simulink model "DragModelSeparateRotors"  (R2015b)
settings: Solver=VariableStepAuto  StartTime=0.0  StopTime=10.0  RelTol=1e-3
settings Model: Creator=jban039  LastModifiedBy=jban039

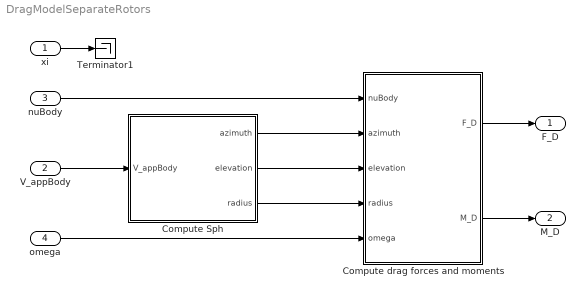
== system DragModelSeparateRotors ==
  xi : Inport  PortDimensions=3
  V_appBody : Inport  Port=2  PortDimensions=3
  nuBody : Inport  Port=3  PortDimensions=3
  omega : Inport  Port=4  PortDimensions=Uav.N_ROTORS
  Compute Sph : MATLAB Function  TreatAsAtomicUnit=on
  Compute drag forces and moments : MATLAB Function  TreatAsAtomicUnit=on
  Terminator1 : Terminator
  F_D : Outport
  M_D : Outport  Port=2
  wires:
  Compute drag forces and moments/1(F_D) -> F_D/1
  Compute drag forces and moments/2(M_D) -> M_D/1
  xi/1 -> Terminator1/1
  omega/1 -> Compute drag forces and moments/5(omega)
  nuBody/1 -> Compute drag forces and moments/1(nuBody)
  V_appBody/1 -> Compute Sph/1(V_appBody)
  Compute Sph/3(radius) -> Compute drag forces and moments/4(radius)
  Compute Sph/2(elevation) -> Compute drag forces and moments/3(elevation)
  Compute Sph/1(azimuth) -> Compute drag forces and moments/2(azimuth)

== matlab function DragModelSeparateRotors/Compute Sph ==
  data: V_appBody input; azimuth output; elevation output; radius output
function [azimuth, elevation, radius] = computeSph(V_appBody)
%#codegen

% Convert from polar to spherical coordinates
[ azimuth, elevation, radius ] = cart2sph( V_appBody(1), V_appBody(2), V_appBody(3) );

== matlab function DragModelSeparateRotors/Compute drag forces and moments ==
  data: nuBody input; azimuth input; elevation input; radius input; omega input; F_D output; M_D output; Uav parameter
function [F_D, M_D] = computeDrag(nuBody, azimuth, elevation, radius, omega, Uav)
%#codegen

% Margin to prevent shattering - doesn't seem to work
% for i = 1:3
%     if ( ( V_appBody(i) > -0.002 ) && ( V_appBody(i) < 0.002 ) )
%         V_appBody(i) = 0;
%     end
% end

% Convert from polar to spherical coordinates
% [ azimuth, elevation, radius ] = cart2sph( V_appBody(1), V_appBody(2), V_appBody(3) );

elevationAbs = abs(elevation);

if ( elevationAbs > pi/4 )
    elevationAbs = pi/4;
end

% A = 0.0381169670063285+...
%     0.00544289693851381   * elevationAbs + ...
%     -1.40320372862409e-05 * mean( omega ) + ...
%     0.0957929844288627    * elevationAbs^2 + ...
%     -3.68966937291996e-05 * elevationAbs * mean( omega ) + ...
%     -5.12058246754513e-08 * mean( omega ).^2;
% B = 2.26155855608694e-05 + ...
%     2.61717004305892e-05 * elevationAbs + ...
%     2.25793855676601e-06 * mean( omega );

A = 1.691827013696288e-01+...
    -1.296810868298392e-01*cos(-elevation)+...
    -6.165562917427734e-05*mean(omega)+...
    1.745617317423599e-05*cos(-elevation)*mean(omega)+...
    1.587622118174535e-08*mean(omega)^2;
B = -2.677662266228434e-01+...
    2.538589720234431e-01*cos(-elevation)+...
    2.743121165911884e-04*mean(omega)+...
    4.813186228167399e-04*cos(-elevation)*mean(omega)+...
    3.930873876708278e-07*mean(omega)^2;

% A  = 3.922073463294323e-02 + 3.047871210062095e-02 * abs(eta(2)) + ...
%    -3.963450428543714e-05 * mean( omega );

% B = 2.261558556086950e-05 + 2.617170043058871e-05 * abs(eta(2)) + ...
%    2.257938556766014e-06 * mean( omega );

% % Calculate linear drag force
% f_D = 0.5 * Uav.RHO_AIR * A * radius^2 + ...
%     0.5 * Uav.RHO_AIR * B * radius * mean(omega);
% F_D = zeros(3,1);

f_D = 0.5 * Uav.RHO_AIR * A * radius^2 + ...
    0.5 * Uav.RHO_AIR * B * radius;
F_D = zeros(3,1);

f_l = 0.5 * Uav.RHO_AIR * -(-3.928287694836059e-02*-elevation+8.917477120052557e-03) * radius^2;
F_l = zeros(3,1);

[ F_D(1), F_D(2), F_D(3) ] = sph2cart( azimuth, elevation, f_D );
[ F_l(1), F_l(2), F_l(3) ] = sph2cart( azimuth, elevation + pi/2, f_l );

F_D = F_D - F_l; 

% Drag moment, applied to independent axes
M_D = 0.5 * Uav.RHO_AIR * Uav.C_DM * ( norm(nuBody) .* nuBody );
